simulink model "RCAMSimulation"  (R2023a)
settings: Solver=VariableStepAuto  StartTime=0.0  StopTime=TF  RelTol=1e-3
values from neighbouring files (symbols this model uses):
  Pos_G0 = [0,0,0]    [Initialize.m]
  u1max = 25*pi/180    (= 0.436332312999)    [Initialize.m]
  u1min = -25*pi/180    (= -0.436332312999)    [Initialize.m]
  u2max = 10*pi/180    (= 0.174532925199)    [Initialize.m]
  u2min = -25*pi/180    (= -0.436332312999)    [Initialize.m]
  u3max = 30*pi/180    (= 0.523598775598)    [Initialize.m]
  u3min = -30*pi/180    (= -0.523598775598)    [Initialize.m]
  u4max = 10*pi/180    (= 0.174532925199)    [Initialize.m]
  u4min = 0*pi/180    (= 0)    [Initialize.m]
  u5max = 10*pi/180    (= 0.174532925199)    [Initialize.m]
  u5min = 0*pi/180    (= 0)    [Initialize.m]
  x0 = [85 ... (first row only)    [Initialize.m]
undefined symbols (not defined in the file or in its folder): RCAM_model
libraries: rllib x1
settings Model: Creator=13911  LastModifiedBy=13911
settings SolverCC: AlgebraicLoopSolver=TrustRegion
settings DataIOCC: ReturnWorkspaceOutputs=off
settings DebuggingCC: UnconnectedInputMsg=warning  UnconnectedOutputMsg=warning  UnconnectedLineMsg=warning  ArithmeticOperatorsInVariantConditions=warning
settings ModelReferenceCC: EnableRefExpFcnMdlSchedulingChecks=on
settings SFSimCC: SimUseLocalCustomCode=off  CustomCodeUndefinedFunction=UseInterfaceOnly
settings RTWCC: RTWUseLocalCustomCode=off
settings CodeAppCC: StateflowObjectComments=on

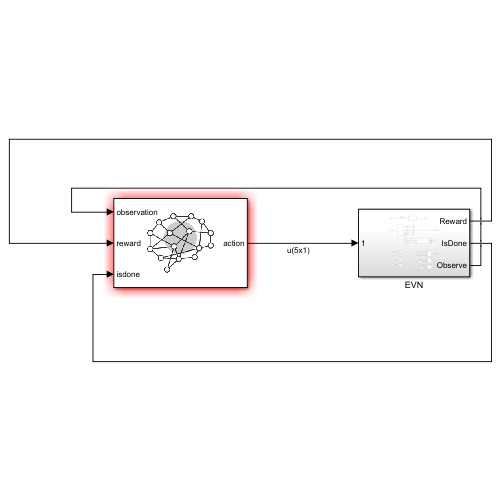
[thumbnail: Simulink's stored preview of the top-level diagram]
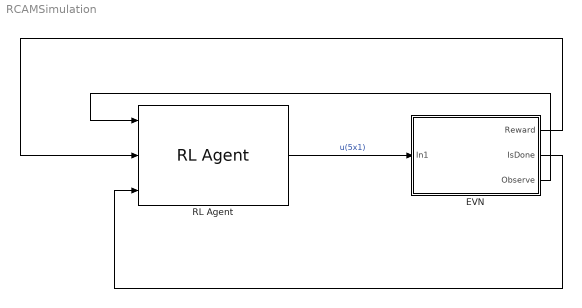
== system RCAMSimulation ==
  EVN : Subsystem
  RL Agent : rllib/RL Agent  Agent=agent_YAG  ExternalActionAsInput=off  ProvideLastAction=off  ProvideCumRwd=off  TreatAsDirectFeedthrough=on  UseStrictObservationDataTypes=off
  wires:
  RL Agent/1 -> EVN/1(In1)  "u(5x1)"
  EVN/1(Reward) -> RL Agent/2
  EVN/2(IsDone) -> RL Agent/3
  EVN/3(Observe) -> RL Agent/1

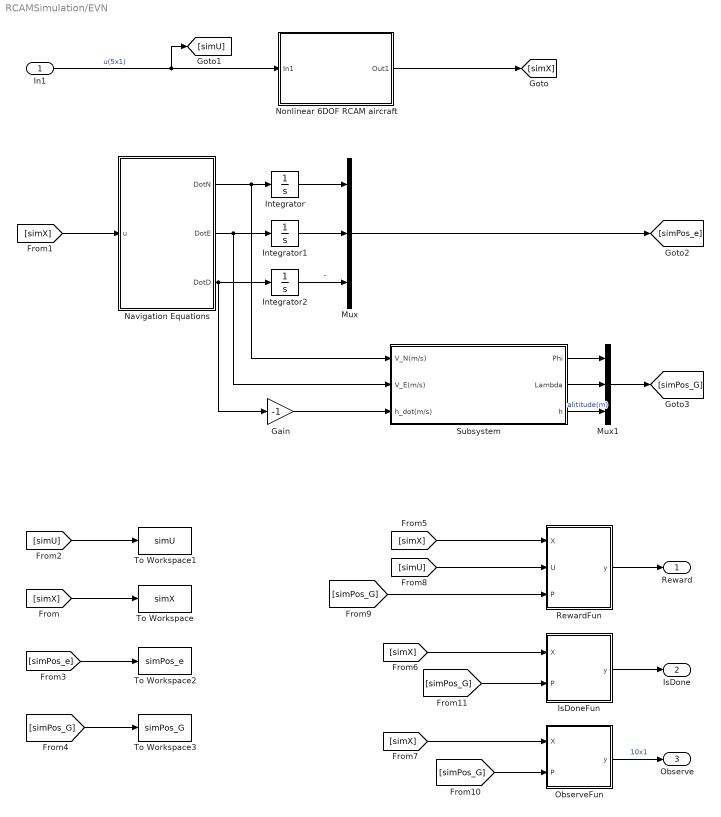
== system RCAMSimulation/EVN ==
  In1 : Inport
  Gain : Gain  Gain=-1
  Integrator : Integrator
  Integrator1 : Integrator
  Integrator2 : Integrator
  IsDoneFun : MATLAB Function  TreatAsAtomicUnit=on
  Mux : Mux  Inputs=3
  Mux1 : Mux  Inputs=3
  Navigation Equations : MATLAB Function  TreatAsAtomicUnit=on
  Nonlinear 6DOF RCAM aircraft : Subsystem
  ObserveFun : MATLAB Function  TreatAsAtomicUnit=on
  RewardFun : MATLAB Function  TreatAsAtomicUnit=on
  Subsystem : Subsystem
  To Workspace : ToWorkspace  VariableName=simX  SaveFormat=Timeseries  SampleTime=-1
  To Workspace1 : ToWorkspace  VariableName=simU  SaveFormat=Timeseries  SampleTime=-1
  To Workspace2 : ToWorkspace  VariableName=simPos_e  SaveFormat=Timeseries  SampleTime=-1
  To Workspace3 : ToWorkspace  VariableName=simPos_G  SaveFormat=Timeseries  SampleTime=-1
  Reward : Outport
  IsDone : Outport  Port=2
  Observe : Outport  Port=3
  wires:
  In1/1 -> Nonlinear 6DOF RCAM aircraft/1(In1), [simU]  "u(5x1)"
  Subsystem/3(h) -> Mux1/3  "alititude(m)"
  Integrator1/1 -> Mux/2
  Navigation Equations/1(DotN) -> Integrator/1, Subsystem/1(V_N(m/s))
  Navigation Equations/2(DotE) -> Integrator1/1, Subsystem/2(V_E(m/s))
  Nonlinear 6DOF RCAM aircraft/1(Out1) -> [simX]
  Integrator/1 -> Mux/1
  Navigation Equations/3(DotD) -> Gain/1, Integrator2/1
  Subsystem/2(Lambda) -> Mux1/2
  Subsystem/1(Phi) -> Mux1/1
  Gain/1 -> Subsystem/3(h_dot(m/s))
  Integrator2/1 -> Mux/3  "-"
  [simX] -> To Workspace/1
  [simX] -> Navigation Equations/1(u)
  [simU] -> To Workspace1/1
  Mux/1 -> [simPos_e]
  [simPos_e] -> To Workspace2/1
  Mux1/1 -> [simPos_G]
  [simPos_G] -> To Workspace3/1
  [simX] -> RewardFun/1(X)
  [simX] -> IsDoneFun/1(X)
  [simX] -> ObserveFun/1(X)
  [simU] -> RewardFun/2(U)
  [simPos_G] -> RewardFun/3(P)
  RewardFun/1(y) -> Reward/1
  IsDoneFun/1(y) -> IsDone/1
  ObserveFun/1(y) -> Observe/1  "10x1"
  [simPos_G] -> ObserveFun/2(P)
  [simPos_G] -> IsDoneFun/2(P)

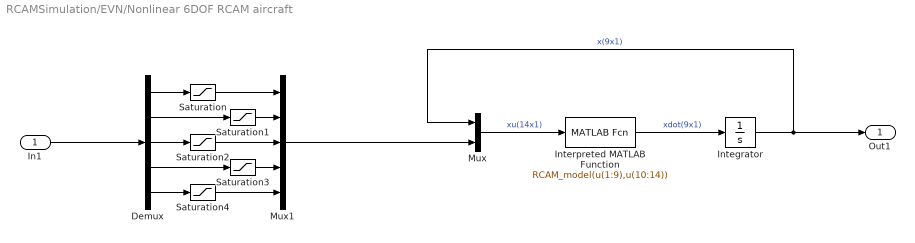
== system RCAMSimulation/EVN/Nonlinear 6DOF RCAM aircraft ==
  In1 : Inport
  Demux : Demux  Outputs=5
  Integrator : Integrator  InitialCondition=x0
  Interpreted MATLAB Function : MATLABFcn  MATLABFcn=RCAM_model(u(1:9),u(10:14))
  Mux : Mux  Inputs=2
  Mux1 : Mux  Inputs=5
  Saturation : Saturate  UpperLimit=u1max  LowerLimit=u1min
  Saturation1 : Saturate  UpperLimit=u2max  LowerLimit=u2min
  Saturation2 : Saturate  UpperLimit=u3max  LowerLimit=u3min
  Saturation3 : Saturate  UpperLimit=u4max  LowerLimit=u4min
  Saturation4 : Saturate  UpperLimit=u5max  LowerLimit=u5min
  Out1 : Outport
  wires:
  Mux/1 -> Interpreted MATLAB Function/1  "xu(14x1)"
  Interpreted MATLAB Function/1 -> Integrator/1  "xdot(9x1)"
  Integrator/1 -> Out1/1, Mux/1  "x(9x1)"
  In1/1 -> Demux/1
  Demux/1 -> Saturation/1
  Demux/2 -> Saturation1/1
  Demux/3 -> Saturation2/1
  Demux/4 -> Saturation3/1
  Demux/5 -> Saturation4/1
  Mux1/1 -> Mux/2
  Saturation/1 -> Mux1/1
  Saturation1/1 -> Mux1/2
  Saturation2/1 -> Mux1/3
  Saturation3/1 -> Mux1/4
  Saturation4/1 -> Mux1/5

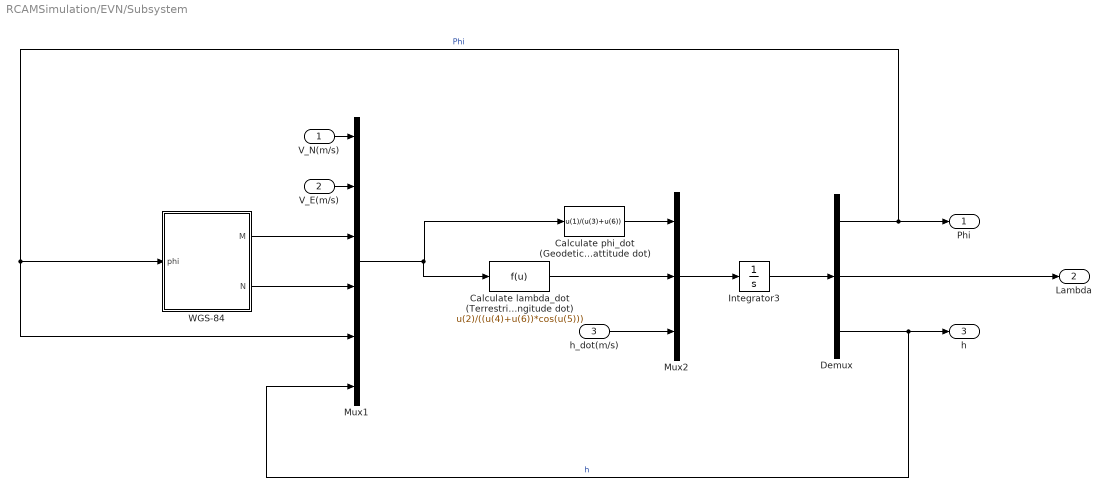
== system RCAMSimulation/EVN/Subsystem ==
  V_N(m/s) : Inport
  V_E(m/s) : Inport  Port=2
  h_dot(m/s) : Inport  Port=3
  Calculate lambda_dot (Terrestrial Longitude dot) : Fcn  Expr=u(2)/((u(4)+u(6))*cos(u(5)))
  Calculate phi_dot (Geodetic Lattitude dot) : Fcn  Expr=u(1)/(u(3)+u(6))
  Demux : Demux  Outputs=3
  Integrator3 : Integrator  InitialCondition=Pos_G0
  Mux1 : Mux  Inputs=6
  Mux2 : Mux  Inputs=3
  WGS-84 : Subsystem
  Phi : Outport
  Lambda : Outport  Port=2
  h : Outport  Port=3
  wires:
  Mux1/1 -> Calculate lambda_dot (Terrestrial Longitude dot)/1, Calculate phi_dot (Geodetic Lattitude dot)/1
  Mux2/1 -> Integrator3/1
  Calculate phi_dot (Geodetic Lattitude dot)/1 -> Mux2/1
  Calculate lambda_dot (Terrestrial Longitude dot)/1 -> Mux2/2
  Integrator3/1 -> Demux/1
  WGS-84/2(N) -> Mux1/4
  WGS-84/1(M) -> Mux1/3
  Demux/2 -> Lambda/1
  V_N(m/s)/1 -> Mux1/1
  Demux/1 -> Mux1/5, WGS-84/1(phi), Phi/1  "Phi"
  Demux/3 -> Mux1/6, h/1  "h"
  V_E(m/s)/1 -> Mux1/2
  h_dot(m/s)/1 -> Mux2/3

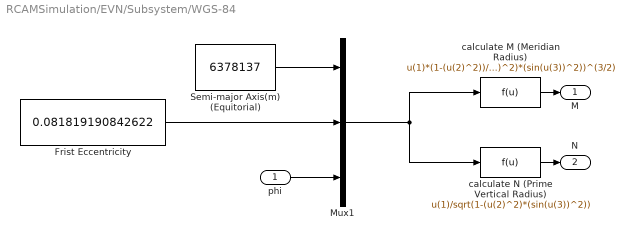
== system RCAMSimulation/EVN/Subsystem/WGS-84 ==
  phi : Inport
  Frist Eccentricity : Constant  Value=0.081819190842622
  Mux1 : Mux  Inputs=3
  Semi-major Axis(m) (Equitorial) : Constant  Value=6378137
  calculate M (Meridian Radius) : Fcn  Expr=u(1)*(1-(u(2)^2))/((1-u(2)^2)*(sin(u(3))^2))^(3/2)
  calculate N (Prime Vertical Radius) : Fcn  Expr=u(1)/sqrt(1-(u(2)^2)*(sin(u(3))^2))
  M : Outport
  N : Outport  Port=2
  wires:
  Semi-major Axis(m) (Equitorial)/1 -> Mux1/1
  calculate N (Prime Vertical Radius)/1 -> N/1
  calculate M (Meridian Radius)/1 -> M/1
  Mux1/1 -> calculate M (Meridian Radius)/1, calculate N (Prime Vertical Radius)/1
  Frist Eccentricity/1 -> Mux1/2
  phi/1 -> Mux1/3

== matlab function RCAMSimulation/EVN/RewardFun ==
  data: X input; y output; U input; P input
function y = fcn(X,U,P)
%% 设计奖励函数
% 目标任务平稳起飞到2000km


%输入惩罚

Reward_U = sum(U.^2);

%状态奖励
Reward_X= sum(X.^2);

%位置奖励
Reward_P = (abs(P(3)-2000)/2000)^2;

y = -Reward_U - Reward_X - Reward_P;

== matlab function RCAMSimulation/EVN/Navigation Equations ==
  data: u input; DotN output; DotE output; DotD output
function [DotN,DotE,DotD] = fcn(u)
x1 = u(1);
x2 = u(2);
x3 = u(3);
x4 = u(4);
x5 = u(5);
x6 = u(6);
x7 = u(7);
x8 = u(8);
x9 = u(9);




c1v = [cos(x9),sin(x9),0;-sin(x9),cos(x9),0;0,0,1];
c21 = [cos(x8),0,-sin(x8);0,1,0;sin(x8),0,cos(x8)];
cb2 = [1,0,0;0,cos(x7),sin(x7);0,-sin(x7),cos(x7)];

cbv = cb2*c21*c1v;
cvb = cbv';
V_b = [x1,x2,x3]';
V_e = cvb*V_b ;
DotN= V_e(1);
DotE= V_e(2);
DotD= V_e(3);

== matlab function RCAMSimulation/EVN/IsDoneFun ==
  data: X input; y output; P input
function y = fcn(X,P)
y = 0;
if P(3) > 4000
    y = 1;
end

% 轴向速度
if X(1)<0 || X(1)>300
    y = 1;
end
% 攻角限制
if X(2)<0 || X(2)>40
    y = 1;
end
% 侧滑角限制
if X(3)<0 || X(3)>40
    y = 1;
end
% 俯仰角限制
if X(7)<-20/57.3 || X(7)>20/57.3
    y = 1;
end
% 滚转角限制
if X(8)<-20/57.3 || X(8)>20/57.3
    y = 1;
end

== matlab function RCAMSimulation/EVN/ObserveFun ==
  data: X input; y output; P input
function y = fcn(X,P)
 y = [X;P(3)];
